simulink model "MSFartoystyring_1_8"  (R2017b)
settings: Solver=ode45  StartTime=tstart  StopTime=tstop  RelTol=1e-3  EnableMultiTasking=on
values from neighbouring files (symbols this model uses):
  c = 0    [analyse_dynamics_v3.m]    (also in analysis_dynamics.m; run.m = 9.87e-06; run_task_1_8.m; solve_diff.m = 0.0007188)
  d_1 = 0.003*10^3    (= 3)    [run_task_1_8.m]
  d_2 = 0.004*10^3    (= 4)    [run_task_1_8.m]
  K_i = lambda^2    [run_task_1_8.m]
  K_p = 2*lambda    [run_task_1_8.m]
  m = 3.5512*10^3    (= 3551.2)    [run_task_1_8.m]
  p0 = zeros(2,1)    [analyse_dynamics_v3.m]    (also in analysis_dynamics.m; run.m; run_task_1_8.m)
  psi0 = 0    [analyse_dynamics_v3.m]    (also in analysis_dynamics.m; run.m; run_task_1_8.m)
  r0 = 0    [analyse_dynamics_v3.m]    (also in analysis_dynamics.m; run.m; run_task_1_8.m)
  tsamp = 100    [analyse_dynamics_v3.m]    (also in analysis_dynamics.m; run.m = 10; run_task_1_8.m = 10)
  u_d = 4    [run_task_1_8.m]
  v0 = [6.63 0]'    [analyse_dynamics_v3.m]    (also in analysis_dynamics.m; run.m; run_task_1_8.m)
undefined symbols (not defined in the file or in its folder): msfartoystyring
settings Model: ExtModeAutoUpdateStatusClock=off  Creator=christh  LastModifiedBy=EllaLovise
settings DataIOCC: LimitDataPoints=on  SaveFormat=Array  SignalLoggingSaveFormat=ModelDataLogs
settings OptimizationCC: ExpressionDepthLimit=2147483647  InitFltsAndDblsToZero=on  LifeSpan=inf
settings DebuggingCC: UnderspecifiedInitializationDetection=Classic  MergeDetectMultiDrivingBlocksExec=none  SolverPrmCheckMsg=warning  FcnCallInpInsideContextMsg=warning  StateNameClashWarn=warning  SFUnexpectedBacktrackingDiag=warning  SFNoUnconditionalDefaultTransitionDiag=warning  SFExecutionAtInitializationDiag=none
settings HardwareCC: ProdBitPerPointer=32  ProdBitPerSizeT=32  ProdBitPerPtrDiffT=32  ProdLargestAtomicFloat=None  ProdIntDivRoundTo=Undefined  ProdEndianess=Unspecified  ProdWordSize=32  ProdHWDeviceType=32-bit Generic
settings ModelReferenceCC: PropagateSignalLabelsOutOfModel=off
settings CodeAppCC: StateflowObjectComments=on
settings GRTTargetCC: TargetLangStandard=C89/C90 (ANSI)  GeneratePreprocessorConditionals=Disable all  CombineOutputUpdateFcns=off  GRTInterface=on
settings ConfigComp: CovMetricSettings=dw  CovHtmlReporting=on  CovSaveCumulativeToWorkspaceVar=on  CovSaveSingleToWorkspaceVar=on  CovExternalEMLEnable=off

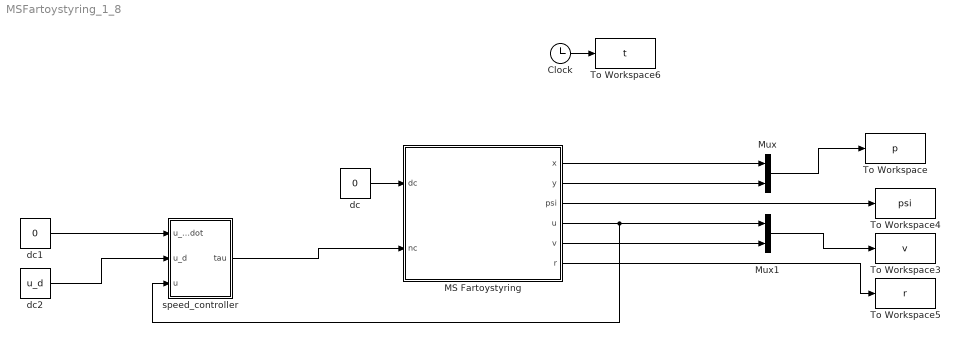
== system MSFartoystyring_1_8 ==
  Clock : Clock
  MS Fartoystyring : Subsystem  mask(MS Fartoystyring for Assignment 3 G&C){x0=p0(1), y0=p0(2), u0=v0(1), v0=v0(2), psi0=psi0, r0=r0, c=c}
      mask prompts: x0 "x(t0) (m)"; y0 "y(t0) (m)"; u0 "u(t0) (m/s)"; v0 "v(t0) (m/s)"; psi0 "psi(t0) (rad)"; r0 "r(t0) (rad/s)"; c "current (0 or 1)"
      mask help:
      | Block corresponding to Figure 1 in the assignment text. Gives the response of the ship.
      |
      | The design speed of MS Fartoystyring is u=8.23 m/s.
      |
      | Input:
      | dc: commanded rudder (rad), dmax=25*pi/180
      | nc: commanded shaft speed (rad/s), nmax=85*2*pi/60
      |
      | Output:
      | x: north pos (m)
      | y: east pos (m)
      | u: surge (m/s)
      | v: sway (m/s)
      | psi: heading (rad)
      | r: yaw (rad/s)
      mask Help: Comments, bugs and help requests can be directed to the TA. Email on course website.
  Mux : Mux  Inputs=2
  Mux1 : Mux  Inputs=2
  To Workspace : ToWorkspace  VariableName=p  SampleTime=tsamp
  To Workspace3 : ToWorkspace  VariableName=v  SampleTime=tsamp
  To Workspace4 : ToWorkspace  VariableName=psi  SampleTime=tsamp
  To Workspace5 : ToWorkspace  VariableName=r  SampleTime=tsamp
  To Workspace6 : ToWorkspace  VariableName=t  SampleTime=tsamp
  dc : Constant  Value=0
  dc1 : Constant  Value=0
  dc2 : Constant  Value=u_d
  speed_controller : Subsystem
  wires:
  Clock/1 -> To Workspace6/1
  MS Fartoystyring/1(x) -> Mux/1
  MS Fartoystyring/2(y) -> Mux/2
  MS Fartoystyring/4(u) -> speed_controller/3(u), Mux1/1
  MS Fartoystyring/5(v) -> Mux1/2
  Mux/1 -> To Workspace/1
  Mux1/1 -> To Workspace3/1
  MS Fartoystyring/3(psi) -> To Workspace4/1
  MS Fartoystyring/6(r) -> To Workspace5/1
  dc/1 -> MS Fartoystyring/1(dc)
  speed_controller/1(tau) -> MS Fartoystyring/2(nc)
  dc1/1 -> speed_controller/1(u_d_dot)
  dc2/1 -> speed_controller/2(u_d)

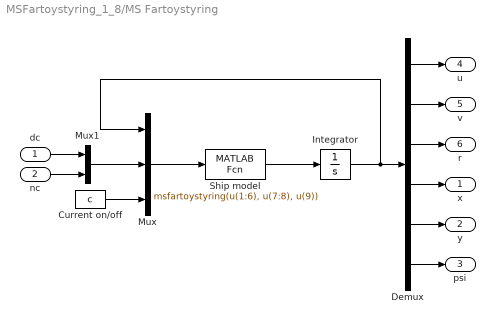
== system MSFartoystyring_1_8/MS Fartoystyring ==
  dc : Inport
  nc : Inport  Port=2
  Current on/off : Constant  Value=c
  Demux : Demux  Outputs=6
  Integrator : Integrator  InitialCondition=[u0 v0 r0 x0 y0 psi0]'
  Mux : Mux  Inputs=3
  Mux1 : Mux  Inputs=2
  Ship model : MATLABFcn  MATLABFcn=msfartoystyring(u(1:6), u(7:8), u(9))  OutputDimensions=6
  x : Outport
  y : Outport  Port=2
  psi : Outport  Port=3
  u : Outport  Port=4
  v : Outport  Port=5
  r : Outport  Port=6
  wires:
  Integrator/1 -> Mux/1, Demux/1
  Mux1/1 -> Mux/2
  dc/1 -> Mux1/1
  nc/1 -> Mux1/2
  Demux/1 -> u/1
  Demux/2 -> v/1
  Demux/3 -> r/1
  Demux/4 -> x/1
  Demux/5 -> y/1
  Demux/6 -> psi/1
  Current on/off/1 -> Mux/3
  Ship model/1 -> Integrator/1
  Mux/1 -> Ship model/1

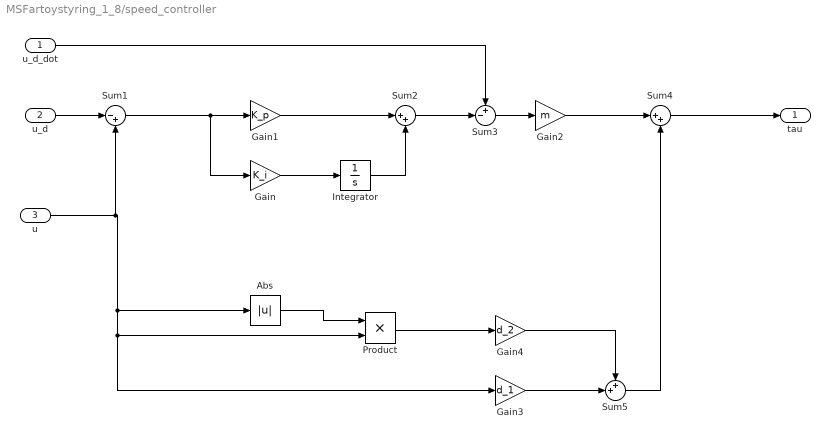
== system MSFartoystyring_1_8/speed_controller ==
  u_d_dot : Inport
  u_d : Inport  Port=2
  u : Inport  Port=3
  Abs : Abs
  Gain : Gain  Gain=K_i
  Gain1 : Gain  Gain=K_p
  Gain2 : Gain  Gain=m
  Gain3 : Gain  Gain=d_1
  Gain4 : Gain  Gain=d_2
  Integrator : Integrator
  Product : Product
  Sum1 : Sum  Inputs=|-+
  Sum2 : Sum  Inputs=|++
  Sum3 : Sum  Inputs=+-|
  Sum4 : Sum  Inputs=|++
  Sum5 : Sum  Inputs=++|
  tau : Outport
  wires:
  Sum1/1 -> Gain/1, Gain1/1
  u/1 -> Gain3/1, Product/2, Abs/1, Sum1/2
  Gain/1 -> Integrator/1
  Sum3/1 -> Gain2/1
  Sum4/1 -> tau/1
  Product/1 -> Gain4/1
  Gain1/1 -> Sum2/1
  Integrator/1 -> Sum2/2
  Gain3/1 -> Sum5/2
  Gain4/1 -> Sum5/1
  Abs/1 -> Product/1
  Sum2/1 -> Sum3/2
  u_d_dot/1 -> Sum3/1
  u_d/1 -> Sum1/1
  Gain2/1 -> Sum4/1
  Sum5/1 -> Sum4/2
